simulink model "TP3"  (R2016b)
settings: Solver=VariableStepAuto  StartTime=0.0  StopTime=10.0  RelTol=1e-3
values from neighbouring files (symbols this model uses):
  a = [0 0 0 8]    [TrabajoPrevio.m]
  b = [0.01 0.7 2 1]    [TrabajoPrevio.m]
  i_v = [15]    [TrabajoPrevio.m]
  step_time = 50    [TrabajoPrevio.m]
  Ts = 0.1    [TrabajoPrevio.m]
libraries: mpclib x1
settings Model: Creator=mariv  LastModifiedBy=mariv

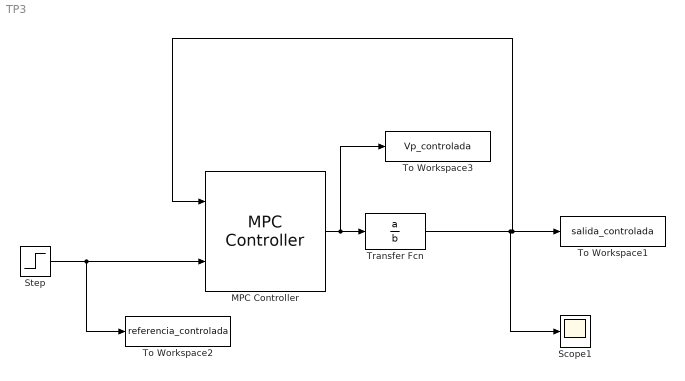
== system TP3 ==
  MPC Controller : mpclib/MPC Controller  SCDEnableBlockLinearizationSpecification=on  mpcobj=mpcobj  is_multiple=0  enable_value=0  return_u0=off  ref_from_ws=off  ref_signal_name=[]  ref_preview=off  md_from_ws=off  md_signal_name=[]  md_preview=off  from_project=off  project_file=MPCtask.mat  md_inport=off  mv_inport=off  cost_outport=off  return_sequence=off  return_qpstatus=off  return_state=off  state_inport=off  lims_inport=off  ywt_inport=off  is_designfromscratch=0  uwt_inport=off  duwt_inport=off  rhoeps_inport=off  uref_inport=off  n_ts=Ts  n_mv=1  n_md=0  n_ud=0  n_mo=1  n_uo=0  BlockDataType=double  SampleTimeInherited=off  switch_inport=off
  Scope1 : Scope
  Step : Step  Time=step_time  Before=i_v  After=step  SampleTime=Ts
  To Workspace1 : ToWorkspace  VariableName=salida_controlada  SaveFormat=Timeseries  SampleTime=-1
  To Workspace2 : ToWorkspace  VariableName=referencia_controlada  SaveFormat=Timeseries  SampleTime=-1
  To Workspace3 : ToWorkspace  VariableName=Vp_controlada  SaveFormat=Timeseries  SampleTime=-1
  Transfer Fcn : TransferFcn  Numerator=a  Denominator=b
  wires:
  Step/1 -> To Workspace2/1, MPC Controller/2
  MPC Controller/1 -> To Workspace3/1, Transfer Fcn/1
  Transfer Fcn/1 -> To Workspace1/1, MPC Controller/1, Scope1/1
